simulink model "fzhomework_tigao"  (R2019a)
settings: Solver=VariableStepAuto  StartTime=0.0  StopTime=10.0  RelTol=1e-3
settings Model: Creator=Administrator  LastModifiedBy=Administrator

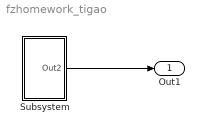
== system fzhomework_tigao ==
  Subsystem : Subsystem  mask{Gain1=3, Gain2=3, Gain3=4, Gain4=5, Gain7=4, Value=pi/3, Gain5=-3, Gain6=-5, InitialCondition2=1, InitialCondition4=0, InitialCondition3=0.5, InitialCondition1=0.2}
      mask prompts: Gain1 "a"; Gain2 "b"; Gain3 "c"; Gain4 "d"; Gain7 "w"; Value "phase"; Gain5 "x1"; Gain6 "x2"; InitialCondition2 "y(0)"; InitialCondition4 "y'(0)"; InitialCondition3 "y''(0)"; InitialCondition1 "y'''(0)"
      mask TypeOptions Gain1: Gain/Gain
      mask TypeOptions Gain2: Gain1/Gain
      mask TypeOptions Gain3: Gain2/Gain
      mask TypeOptions Gain4: Gain3/Gain
      mask TypeOptions Gain7: Gain6/Gain
      mask TypeOptions Value: Constant/Value
      mask TypeOptions Gain5: Gain4/Gain
      mask TypeOptions Gain6: Gain5/Gain
      mask TypeOptions InitialCondition2: Integrator3/InitialCondition
      mask TypeOptions InitialCondition4: Integrator1/InitialCondition
      mask TypeOptions InitialCondition3: Integrator2/InitialCondition
      mask TypeOptions InitialCondition1:
      | Intergrator0
      | /InitialCondition
  Out1 : Outport
  wires:
  Subsystem/1(Out2) -> Out1/1

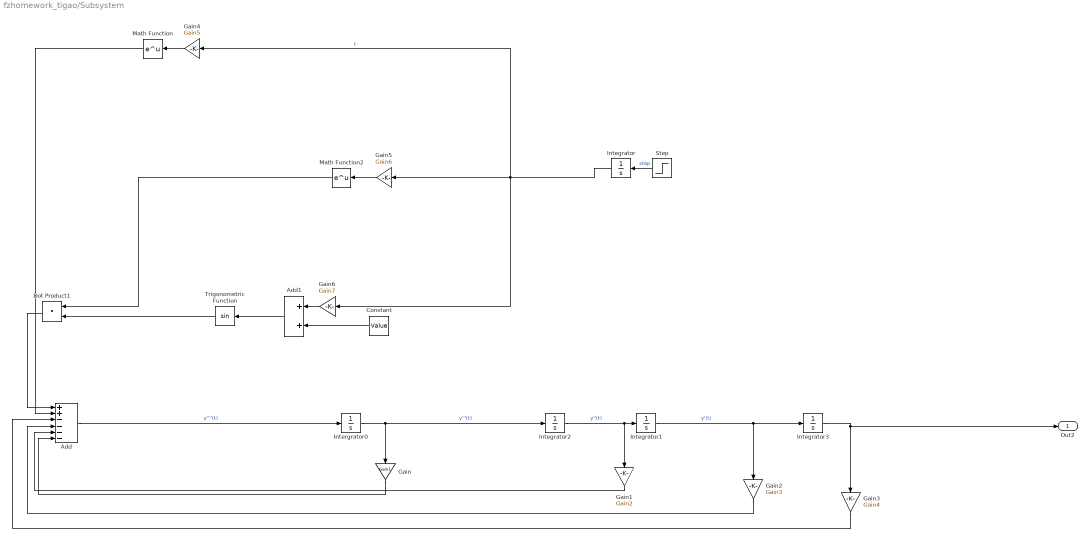
== system fzhomework_tigao/Subsystem ==
  Add : Sum  Inputs=++----
  Add1 : Sum
  Constant : Constant  Value=Value
  Dot Product1 : DotProduct  InputSameDT=on  OutDataTypeStr=Inherit: Inherit via internal rule
  Gain : Gain  Gain=Gain1
  Gain1 : Gain  Gain=Gain2
  Gain2 : Gain  Gain=Gain3
  Gain3 : Gain  Gain=Gain4
  Gain4 : Gain  Gain=Gain5
  Gain5 : Gain  Gain=Gain6
  Gain6 : Gain  Gain=Gain7
  Integrator : Integrator
  Integrator1 : Integrator  InitialCondition=InitialCondition4
  Integrator2 : Integrator  InitialCondition=InitialCondition3
  Integrator3 : Integrator  InitialCondition=InitialCondition2
  "Intergrator0 " : Integrator  InitialCondition=InitialCondition1
  Math Function : Math  SaturateOnIntegerOverflow=on
  Math Function2 : Math  SaturateOnIntegerOverflow=on
  Step : Step  SampleTime=0
  Trigonometric Function : Trigonometry
  Out2 : Outport
  wires:
  Add/1 -> "Intergrator0 "/1  "y''''(t)"
  Gain2/1 -> Add/4
  Dot Product1/1 -> Add/1
  Integrator2/1 -> Gain1/1, Integrator1/1  "y''(t)"
  Gain1/1 -> Add/5
  Trigonometric Function/1 -> Dot Product1/2
  Constant/1 -> Add1/2
  Gain4/1 -> Math Function/1
  Gain/1 -> Add/6
  Math Function/1 -> Add/2
  "Intergrator0 "/1 -> Gain/1, Integrator2/1  "y'''(t)"
  Integrator1/1 -> Integrator3/1, Gain2/1  "y'(t)"
  Gain6/1 -> Add1/1
  Add1/1 -> Trigonometric Function/1
  Gain3/1 -> Add/3
  Integrator3/1 -> Out2/1, Gain3/1
  Math Function2/1 -> Dot Product1/1
  Gain5/1 -> Math Function2/1
  Integrator/1 -> Gain4/1, Gain6/1, Gain5/1  "t"
  Step/1 -> Integrator/1  "step"
